simulink library "AfsSlaveLib"  (R2020b)
settings: Solver=VariableStepAuto  StartTime=0.0  StopTime=10.0  RelTol=1e-3
libraries: Ramp_Library_R2017b x3, simulink x2
Description:
  | VLS Standard Library
  | Version: 1.0.0
settings Model: Creator=mchawa  LastModifiedBy=ahashem
settings DataIOCC: ReturnWorkspaceOutputs=off
settings DebuggingCC: ArithmeticOperatorsInVariantConditions=warning
settings SFSimCC: SimUseLocalCustomCode=off  CustomCodeUndefinedFunction=UseInterfaceOnly
settings RTWCC: RTWUseLocalCustomCode=off

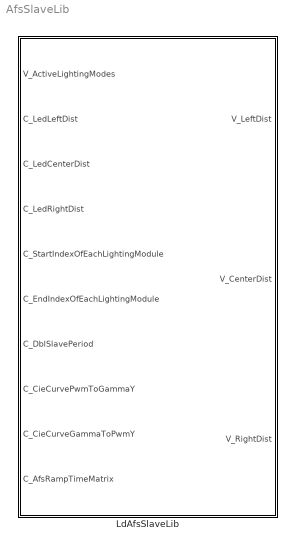
== system AfsSlaveLib ==
  LdAfsSlaveLib : Subsystem  TreatAsAtomicUnit=on

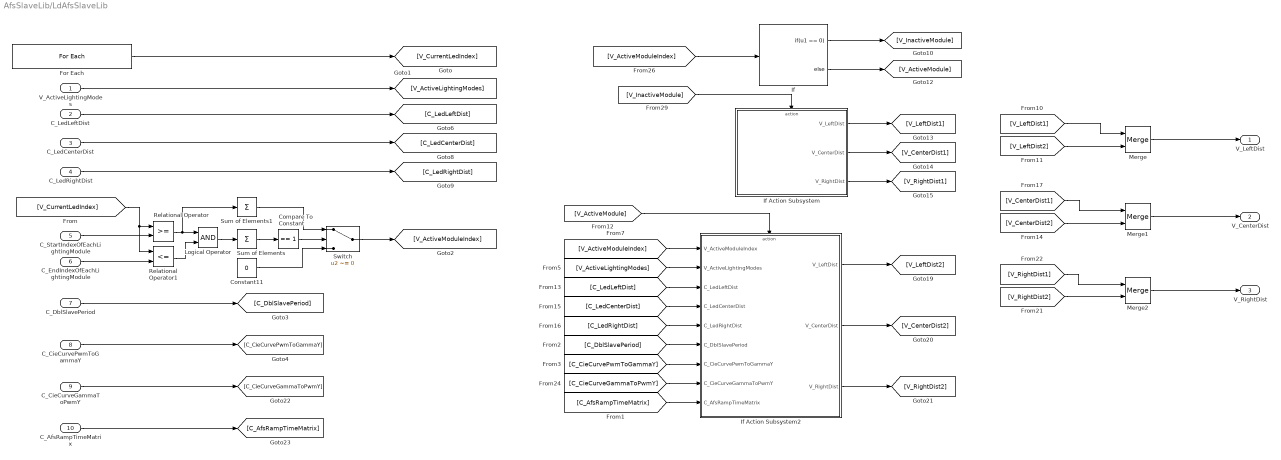
== system AfsSlaveLib/LdAfsSlaveLib ==
  V_ActiveLightingModes : Inport
  C_LedLeftDist : Inport  Port=2  Partition=on  PartitionDimension=2  PartitionWidth=1  PartitionOffset=0
  C_LedCenterDist : Inport  Port=3  Partition=on  PartitionDimension=2  PartitionWidth=1  PartitionOffset=0
  C_LedRightDist : Inport  Port=4  Partition=on  PartitionDimension=2  PartitionWidth=1  PartitionOffset=0
  C_StartIndexOfEachLightingModule : Inport  Port=5
  C_EndIndexOfEachLightingModule : Inport  Port=6
  C_DblSlavePeriod : Inport  Port=7
  C_CieCurvePwmToGammaY : Inport  Port=8
  C_CieCurveGammaToPwmY : Inport  Port=9
  C_AfsRampTimeMatrix : Inport  Port=10
  Compare To Constant : simulink/Logic and Bit Operations/Compare To Constant  relop===  const=1  OutDataTypeStr=boolean
  Constant11 : Constant  Value=0  OutDataTypeStr=Inherit: Inherit via back propagation
  For Each : ForEach  DisableCoverage=on  ShowIterationIndex=on
  If : If  IfExpression=u1 == 0
  If Action Subsystem : Subsystem  TreatAsAtomicUnit=on
  If Action Subsystem2 : Subsystem  TreatAsAtomicUnit=on
  Logical Operator : Logic  AllPortsSameDT=off  OutDataTypeStr=boolean
  Merge : Merge
  Merge1 : Merge
  Merge2 : Merge
  Relational Operator : RelationalOperator  OutDataTypeStr=boolean  RndMeth=Simplest
  Relational Operator1 : RelationalOperator  Operator=<=  OutDataTypeStr=boolean  RndMeth=Simplest
  Sum of Elements : Sum  Inputs=+
  Sum of Elements1 : Sum  Inputs=+
  Switch : Switch  Criteria=u2 ~= 0
  V_LeftDist : Outport  ConcatenationDimension=1  VectorParamsAs1DForOutWhenUnconnected=off
  V_CenterDist : Outport  Port=2  ConcatenationDimension=1  VectorParamsAs1DForOutWhenUnconnected=off
  V_RightDist : Outport  Port=3  ConcatenationDimension=1  VectorParamsAs1DForOutWhenUnconnected=off
  wires:
  Sum of Elements1/1 -> Switch/1
  Constant11/1 -> Switch/3
  Relational Operator1/1 -> Logical Operator/2
  C_StartIndexOfEachLightingModule/1 -> Relational Operator/2
  Relational Operator/1 -> Sum of Elements1/1, Logical Operator/1
  Switch/1 -> [V_ActiveModuleIndex]
  Logical Operator/1 -> Sum of Elements/1
  Compare To Constant/1 -> Switch/2
  C_EndIndexOfEachLightingModule/1 -> Relational Operator1/2
  [V_CurrentLedIndex] -> Relational Operator1/1, Relational Operator/1
  For Each/1 -> [V_CurrentLedIndex]
  V_ActiveLightingModes/1 -> [V_ActiveLightingModes]
  Sum of Elements/1 -> Compare To Constant/1
  If/1 -> [V_InactiveModule]
  [V_ActiveModuleIndex] -> If/1
  If/2 -> [V_ActiveModule]
  [V_InactiveModule] -> If Action Subsystem/Action
  [V_ActiveModule] -> If Action Subsystem2/Action
  Merge/1 -> V_LeftDist/1
  Merge1/1 -> V_CenterDist/1
  Merge2/1 -> V_RightDist/1
  If Action Subsystem/1(V_LeftDist) -> [V_LeftDist1]
  If Action Subsystem/2(V_CenterDist) -> [V_CenterDist1]
  If Action Subsystem/3(V_RightDist) -> [V_RightDist1]
  If Action Subsystem2/1(V_LeftDist) -> [V_LeftDist2]
  If Action Subsystem2/2(V_CenterDist) -> [V_CenterDist2]
  If Action Subsystem2/3(V_RightDist) -> [V_RightDist2]
  [V_LeftDist2] -> Merge/2
  [V_LeftDist1] -> Merge/1
  [V_CenterDist2] -> Merge1/2
  [V_CenterDist1] -> Merge1/1
  [V_RightDist2] -> Merge2/2
  [V_RightDist1] -> Merge2/1
  [V_ActiveLightingModes] -> If Action Subsystem2/2(V_ActiveLightingModes)
  [V_ActiveModuleIndex] -> If Action Subsystem2/1(V_ActiveModuleIndex)
  C_LedCenterDist/1 -> [C_LedCenterDist]
  C_LedRightDist/1 -> [C_LedRightDist]
  C_LedLeftDist/1 -> [C_LedLeftDist]
  [C_LedLeftDist] -> If Action Subsystem2/3(C_LedLeftDist)
  [C_LedCenterDist] -> If Action Subsystem2/4(C_LedCenterDist)
  [C_LedRightDist] -> If Action Subsystem2/5(C_LedRightDist)
  C_DblSlavePeriod/1 -> [C_DblSlavePeriod]
  C_AfsRampTimeMatrix/1 -> [C_AfsRampTimeMatrix]
  C_CieCurveGammaToPwmY/1 -> [C_CieCurveGammaToPwmY]
  C_CieCurvePwmToGammaY/1 -> [C_CieCurvePwmToGammaY]
  [C_DblSlavePeriod] -> If Action Subsystem2/6(C_DblSlavePeriod)
  [C_CieCurvePwmToGammaY] -> If Action Subsystem2/7(C_CieCurvePwmToGammaY)
  [C_CieCurveGammaToPwmY] -> If Action Subsystem2/8(C_CieCurveGammaToPwmY)
  [C_AfsRampTimeMatrix] -> If Action Subsystem2/9(C_AfsRampTimeMatrix)

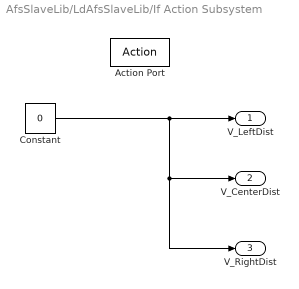
== system AfsSlaveLib/LdAfsSlaveLib/If Action Subsystem ==
  Action Port : ActionPort
  Constant : Constant  Value=0  OutDataTypeStr=Inherit: Inherit via back propagation
  V_LeftDist : Outport  VectorParamsAs1DForOutWhenUnconnected=off
  V_CenterDist : Outport  Port=2  VectorParamsAs1DForOutWhenUnconnected=off
  V_RightDist : Outport  Port=3  VectorParamsAs1DForOutWhenUnconnected=off
  wires:
  Constant/1 -> V_CenterDist/1, V_RightDist/1, V_LeftDist/1

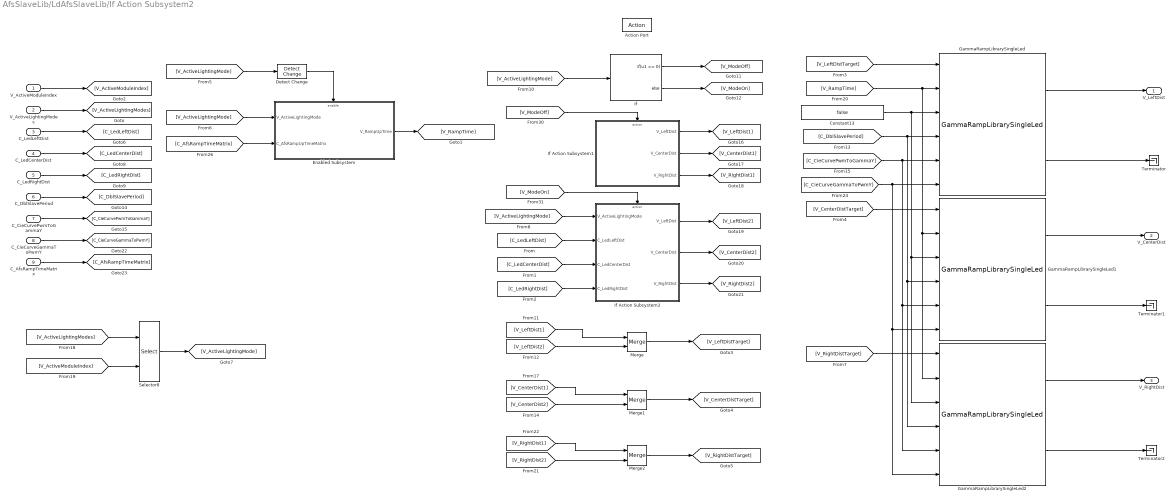
== system AfsSlaveLib/LdAfsSlaveLib/If Action Subsystem2 ==
  V_ActiveModuleIndex : Inport
  V_ActiveLightingModes : Inport  Port=2
  C_LedLeftDist : Inport  Port=3
  C_LedCenterDist : Inport  Port=4
  C_LedRightDist : Inport  Port=5
  C_DblSlavePeriod : Inport  Port=6
  C_CieCurvePwmToGammaY : Inport  Port=7
  C_CieCurveGammaToPwmY : Inport  Port=8
  C_AfsRampTimeMatrix : Inport  Port=9
  Action Port : ActionPort
  Constant13 : Constant  Value=false  OutDataTypeStr=boolean
  Detect Change : simulink/Logic and Bit Operations/Detect Change  vinit=0  OutDataTypeStr=boolean
  Enabled Subsystem : Subsystem  TreatAsAtomicUnit=on
  GammaRampLibrarySingleLed : Ramp_Library_R2017b/GammaRampLibrarySingleLed  Description=|  SystemSampleTime=-1  VariantActivationTime=update diagram  Latency=0  AutoFrameSizeCalculation=off
      | This library performs ramp function taking CIE curves which are evenly distributed.
      | It performs the ramp linearly on the Gamma Curve.
  GammaRampLibrarySingleLed1 : Ramp_Library_R2017b/GammaRampLibrarySingleLed  Description=|  SystemSampleTime=-1  VariantActivationTime=update diagram  Latency=0  AutoFrameSizeCalculation=off
      | This library performs ramp function taking CIE curves which are evenly distributed.
      | It performs the ramp linearly on the Gamma Curve.
  GammaRampLibrarySingleLed2 : Ramp_Library_R2017b/GammaRampLibrarySingleLed  Description=|  SystemSampleTime=-1  VariantActivationTime=update diagram  Latency=0  AutoFrameSizeCalculation=off
      | This library performs ramp function taking CIE curves which are evenly distributed.
      | It performs the ramp linearly on the Gamma Curve.
  If : If  IfExpression=u1 == 0
  If Action Subsystem1 : Subsystem  TreatAsAtomicUnit=on
  If Action Subsystem2 : Subsystem  TreatAsAtomicUnit=on
  Merge : Merge
  Merge1 : Merge
  Merge2 : Merge
  Selector8 : Selector  IndexOptions=Index vector (port)  Indices=[1 3]  OutputSizes=1
  Terminator : Terminator
  Terminator1 : Terminator
  Terminator2 : Terminator
  V_LeftDist : Outport  VectorParamsAs1DForOutWhenUnconnected=off
  V_CenterDist : Outport  Port=2  VectorParamsAs1DForOutWhenUnconnected=off
  V_RightDist : Outport  Port=3  VectorParamsAs1DForOutWhenUnconnected=off
  wires:
  V_ActiveLightingModes/1 -> [V_ActiveLightingModes]
  Selector8/1 -> [V_ActiveLightingMode]
  [V_ActiveLightingModes] -> Selector8/1
  [V_ActiveModuleIndex] -> Selector8/2
  If Action Subsystem2/1(V_LeftDist) -> [V_LeftDist2]
  If Action Subsystem1/3(V_RightDist) -> [V_RightDist1]
  If Action Subsystem1/1(V_LeftDist) -> [V_LeftDist1]
  If Action Subsystem2/3(V_RightDist) -> [V_RightDist2]
  [V_ModeOff] -> If Action Subsystem1/Action
  If Action Subsystem1/2(V_CenterDist) -> [V_CenterDist1]
  [V_ModeOn] -> If Action Subsystem2/Action
  If Action Subsystem2/2(V_CenterDist) -> [V_CenterDist2]
  If/2 -> [V_ModeOn]
  [V_ActiveLightingMode] -> If/1
  If/1 -> [V_ModeOff]
  [V_ActiveLightingMode] -> If Action Subsystem2/1(V_ActiveLightingMode)
  [V_RightDist1] -> Merge2/1
  [V_LeftDist2] -> Merge/2
  [V_CenterDist2] -> Merge1/2
  [V_CenterDist1] -> Merge1/1
  [V_RightDist2] -> Merge2/2
  [V_LeftDist1] -> Merge/1
  V_ActiveModuleIndex/1 -> [V_ActiveModuleIndex]
  Merge/1 -> [V_LeftDistTarget]
  Merge1/1 -> [V_CenterDistTarget]
  Merge2/1 -> [V_RightDistTarget]
  GammaRampLibrarySingleLed/1 -> V_LeftDist/1
  GammaRampLibrarySingleLed1/1 -> V_CenterDist/1
  GammaRampLibrarySingleLed2/1 -> V_RightDist/1
  GammaRampLibrarySingleLed/2 -> Terminator/1
  GammaRampLibrarySingleLed1/2 -> Terminator1/1
  GammaRampLibrarySingleLed2/2 -> Terminator2/1
  C_LedRightDist/1 -> [C_LedRightDist]
  C_LedCenterDist/1 -> [C_LedCenterDist]
  C_LedLeftDist/1 -> [C_LedLeftDist]
  [C_LedLeftDist] -> If Action Subsystem2/2(C_LedLeftDist)
  [C_LedCenterDist] -> If Action Subsystem2/3(C_LedCenterDist)
  [C_LedRightDist] -> If Action Subsystem2/4(C_LedRightDist)
  [V_ActiveLightingMode] -> Detect Change/1
  Detect Change/1 -> Enabled Subsystem/Enable
  [V_ActiveLightingMode] -> Enabled Subsystem/1(V_ActiveLightingMode)
  Enabled Subsystem/1(V_RampUpTime) -> [V_RampTime]
  [V_LeftDistTarget] -> GammaRampLibrarySingleLed/1
  [C_CieCurveGammaToPwmY] -> GammaRampLibrarySingleLed/6, GammaRampLibrarySingleLed2/6, GammaRampLibrarySingleLed1/6
  [C_CieCurvePwmToGammaY] -> GammaRampLibrarySingleLed/5, GammaRampLibrarySingleLed2/5, GammaRampLibrarySingleLed1/5
  [C_DblSlavePeriod] -> GammaRampLibrarySingleLed/4, GammaRampLibrarySingleLed2/4, GammaRampLibrarySingleLed1/4
  Constant13/1 -> GammaRampLibrarySingleLed/3, GammaRampLibrarySingleLed2/3, GammaRampLibrarySingleLed1/3
  [V_RampTime] -> GammaRampLibrarySingleLed2/2, GammaRampLibrarySingleLed1/2, GammaRampLibrarySingleLed/2
  [V_CenterDistTarget] -> GammaRampLibrarySingleLed1/1
  [V_RightDistTarget] -> GammaRampLibrarySingleLed2/1
  C_DblSlavePeriod/1 -> [C_DblSlavePeriod]
  C_CieCurvePwmToGammaY/1 -> [C_CieCurvePwmToGammaY]
  C_CieCurveGammaToPwmY/1 -> [C_CieCurveGammaToPwmY]
  C_AfsRampTimeMatrix/1 -> [C_AfsRampTimeMatrix]
  [C_AfsRampTimeMatrix] -> Enabled Subsystem/2(C_AfsRampUpTimeMatrix)

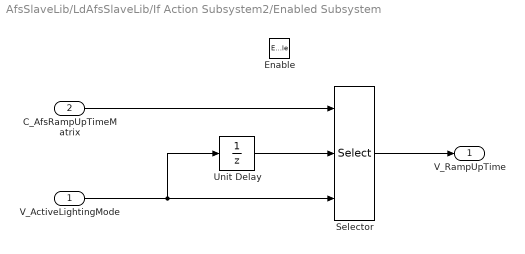
== system AfsSlaveLib/LdAfsSlaveLib/If Action Subsystem2/Enabled Subsystem ==
  V_ActiveLightingMode : Inport
  C_AfsRampUpTimeMatrix : Inport  Port=2
  Enable : EnablePort
  Selector : Selector  NumberOfDimensions=2  IndexMode=Zero-based  InputPortWidth=3  IndexOptions=Index vector (port),Index vector (port)  Indices=[1 3],1  OutputSizes=1,1
  Unit Delay : UnitDelay  SampleTime=-1  HasFrameUpgradeWarning=on
  V_RampUpTime : Outport
  wires:
  Unit Delay/1 -> Selector/2
  Selector/1 -> V_RampUpTime/1
  C_AfsRampUpTimeMatrix/1 -> Selector/1
  V_ActiveLightingMode/1 -> Unit Delay/1, Selector/3

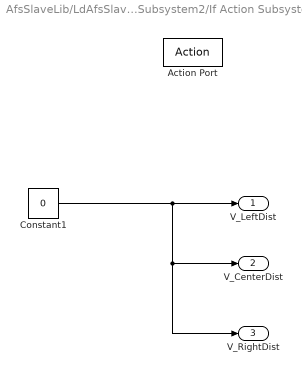
== system AfsSlaveLib/LdAfsSlaveLib/If Action Subsystem2/If Action Subsystem1 ==
  Action Port : ActionPort
  Constant1 : Constant  Value=0  OutDataTypeStr=Inherit: Inherit via back propagation
  V_LeftDist : Outport  VectorParamsAs1DForOutWhenUnconnected=off
  V_CenterDist : Outport  Port=2  VectorParamsAs1DForOutWhenUnconnected=off
  V_RightDist : Outport  Port=3  VectorParamsAs1DForOutWhenUnconnected=off
  wires:
  Constant1/1 -> V_CenterDist/1, V_RightDist/1, V_LeftDist/1

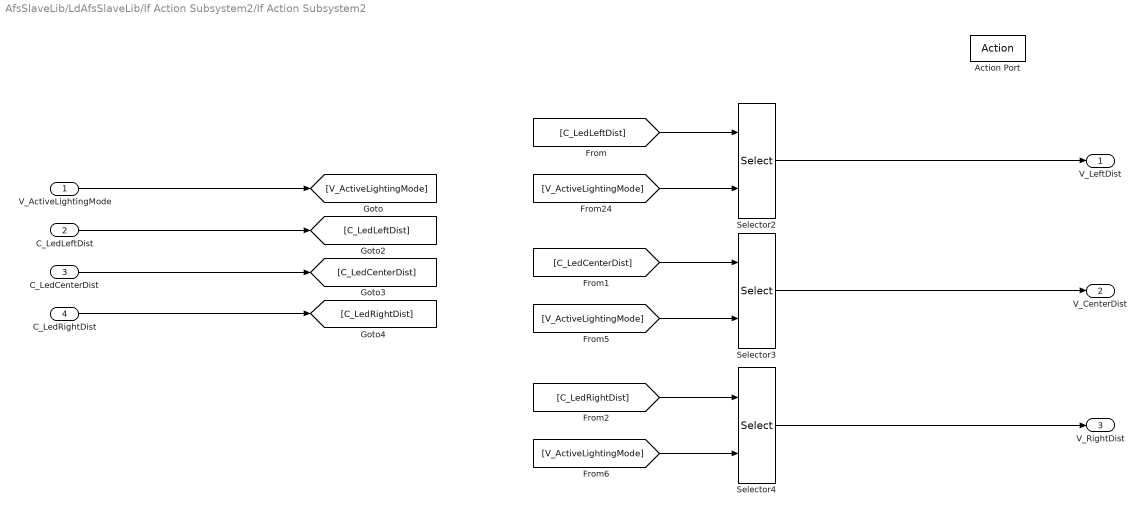
== system AfsSlaveLib/LdAfsSlaveLib/If Action Subsystem2/If Action Subsystem2 ==
  V_ActiveLightingMode : Inport
  C_LedLeftDist : Inport  Port=2
  C_LedCenterDist : Inport  Port=3
  C_LedRightDist : Inport  Port=4
  Action Port : ActionPort
  Selector2 : Selector  NumberOfDimensions=2  InputPortWidth=2  IndexOptions=Index vector (port),Select all  Indices=[1 3],1  OutputSizes=1,1
  Selector3 : Selector  NumberOfDimensions=2  InputPortWidth=2  IndexOptions=Index vector (port),Select all  Indices=[1 3],1  OutputSizes=1,1
  Selector4 : Selector  NumberOfDimensions=2  InputPortWidth=2  IndexOptions=Index vector (port),Select all  Indices=[1 3],1  OutputSizes=1,1
  V_LeftDist : Outport  VectorParamsAs1DForOutWhenUnconnected=off
  V_CenterDist : Outport  Port=2  VectorParamsAs1DForOutWhenUnconnected=off
  V_RightDist : Outport  Port=3  VectorParamsAs1DForOutWhenUnconnected=off
  wires:
  [V_ActiveLightingMode] -> Selector4/2
  [V_ActiveLightingMode] -> Selector2/2
  [V_ActiveLightingMode] -> Selector3/2
  V_ActiveLightingMode/1 -> [V_ActiveLightingMode]
  Selector2/1 -> V_LeftDist/1
  Selector3/1 -> V_CenterDist/1
  Selector4/1 -> V_RightDist/1
  C_LedLeftDist/1 -> [C_LedLeftDist]
  [C_LedLeftDist] -> Selector2/1
  C_LedCenterDist/1 -> [C_LedCenterDist]
  [C_LedCenterDist] -> Selector3/1
  C_LedRightDist/1 -> [C_LedRightDist]
  [C_LedRightDist] -> Selector4/1
